simulink model "linearSim"  (R2021b)
settings: Solver=ode23s  StartTime=0.0  StopTime=50  MaxStep=0.01  RelTol=1e-3
undefined symbols (not defined in the file or in its folder): FE, IRL, P, PE, SE
settings Model: Creator=rushik  LastModifiedBy=rushik
settings DataIOCC: SaveOutput=off  DSMLogging=off  SaveTime=off  ReturnWorkspaceOutputs=off

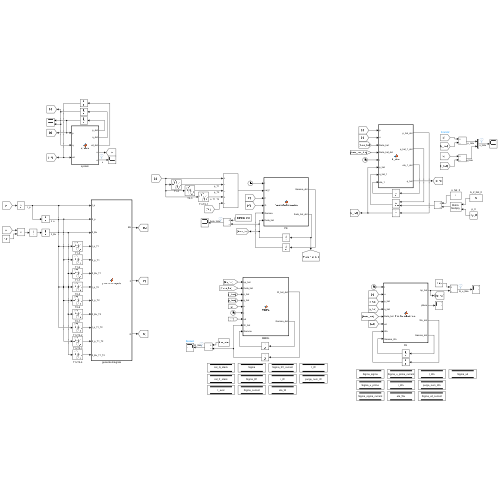
[thumbnail: Simulink's stored preview of the top-level diagram]
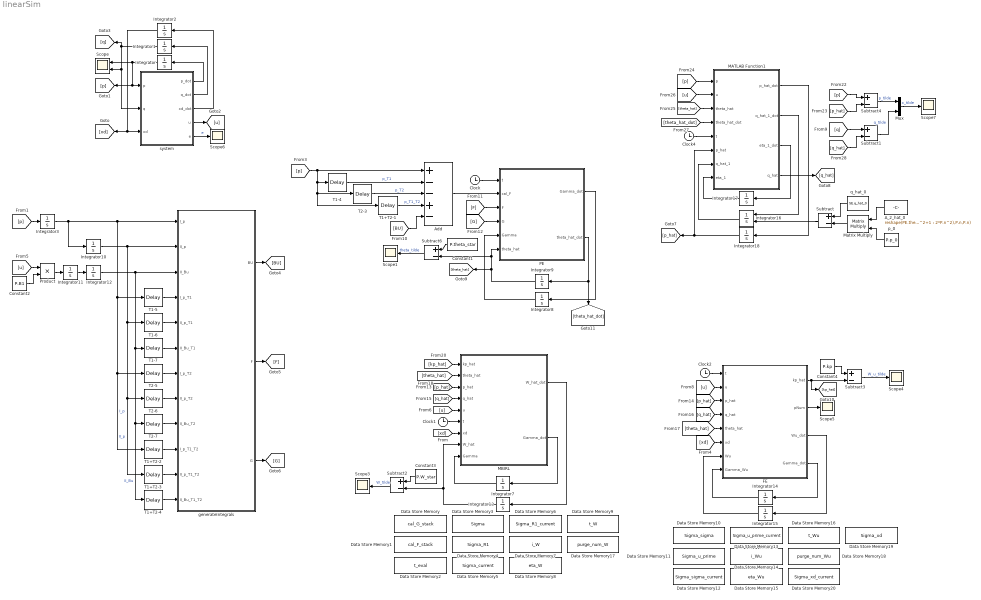
== system linearSim ==
  A_2_hat_0 : Constant  Value=reshape(PE.theta_hat_0(P.n^2+1 : 2*P.n^2),P.n,P.n)
  Add : Sum  Inputs=+--+-
  Clock{,1..2,4} (4 alike) : Clock
  Constant1 : Constant  Value=P.theta_star
  Constant2 : Constant  Value=P.B1
  Constant3 : Constant  Value=P.W_star  VectorParams1D=off
  Constant4 : Constant  Value=P.kp
  Data Store Memory : DataStoreMemory  DataStoreName=cal_G_stack  ReadBeforeWriteMsg=warning  WriteAfterWriteMsg=warning  WriteAfterReadMsg=warning  InitialValue=zeros(2*P.n^2,P.n*PE.N)  VectorParams1D=off  ShowAdditionalParam=off  OutDataTypeStr=double
  Data Store Memory1 : DataStoreMemory  DataStoreName=cal_F_stack  ReadBeforeWriteMsg=warning  WriteAfterWriteMsg=warning  WriteAfterReadMsg=warning  InitialValue=zeros(P.n,PE.N)  VectorParams1D=off  ShowAdditionalParam=off  OutDataTypeStr=double
  Data Store Memory10 : DataStoreMemory  DataStoreName=Sigma_sigma  ReadBeforeWriteMsg=warning  WriteAfterWriteMsg=warning  WriteAfterReadMsg=warning  InitialValue=zeros(FE.M,FE.K)  VectorParams1D=off  ShowAdditionalParam=off  OutDataTypeStr=double
  Data Store Memory11 : DataStoreMemory  DataStoreName=Sigma_u_prime  ReadBeforeWriteMsg=warning  WriteAfterWriteMsg=warning  WriteAfterReadMsg=warning  InitialValue=zeros(FE.M,P.m)  VectorParams1D=off  ShowAdditionalParam=off  OutDataTypeStr=double
  Data Store Memory12 : DataStoreMemory  DataStoreName=Sigma_sigma_current  ReadBeforeWriteMsg=warning  WriteAfterWriteMsg=warning  WriteAfterReadMsg=warning  InitialValue=zeros(FE.M,FE.K)  VectorParams1D=off  ShowAdditionalParam=off  OutDataTypeStr=double
  Data Store Memory13 : DataStoreMemory  DataStoreName=Sigma_u_prime_current  ReadBeforeWriteMsg=warning  WriteAfterWriteMsg=warning  WriteAfterReadMsg=warning  InitialValue=zeros(FE.M,P.m)  VectorParams1D=off  ShowAdditionalParam=off  OutDataTypeStr=double
  Data Store Memory14 : DataStoreMemory  DataStoreName=i_Wu  ReadBeforeWriteMsg=warning  WriteAfterWriteMsg=warning  WriteAfterReadMsg=warning  InitialValue=1  VectorParams1D=off  ShowAdditionalParam=off  OutDataTypeStr=double
  Data Store Memory15 : DataStoreMemory  DataStoreName=eta_Wu  ReadBeforeWriteMsg=warning  WriteAfterWriteMsg=warning  WriteAfterReadMsg=warning  VectorParams1D=off  ShowAdditionalParam=off  OutDataTypeStr=double
  Data Store Memory16 : DataStoreMemory  DataStoreName=t_Wu  ReadBeforeWriteMsg=warning  WriteAfterWriteMsg=warning  WriteAfterReadMsg=warning  VectorParams1D=off  ShowAdditionalParam=off  OutDataTypeStr=double
  Data Store Memory17 : DataStoreMemory  DataStoreName=purge_num_W  ReadBeforeWriteMsg=warning  WriteAfterWriteMsg=warning  WriteAfterReadMsg=warning  VectorParams1D=off  ShowAdditionalParam=off  OutDataTypeStr=double
  Data Store Memory18 : DataStoreMemory  DataStoreName=purge_num_Wu  ReadBeforeWriteMsg=warning  WriteAfterWriteMsg=warning  WriteAfterReadMsg=warning  VectorParams1D=off  ShowAdditionalParam=off  OutDataTypeStr=double
  Data Store Memory19 : DataStoreMemory  DataStoreName=Sigma_xd  ReadBeforeWriteMsg=warning  WriteAfterWriteMsg=warning  WriteAfterReadMsg=warning  InitialValue=zeros(PE.L,FE.M)  VectorParams1D=off  ShowAdditionalParam=off  OutDataTypeStr=double
  Data Store Memory2 : DataStoreMemory  DataStoreName=t_eval  ReadBeforeWriteMsg=warning  WriteAfterWriteMsg=warning  WriteAfterReadMsg=warning  VectorParams1D=off  ShowAdditionalParam=off  OutDataTypeStr=double
  Data Store Memory20 : DataStoreMemory  DataStoreName=Sigma_xd_current  ReadBeforeWriteMsg=warning  WriteAfterWriteMsg=warning  WriteAfterReadMsg=warning  InitialValue=zeros(PE.L,FE.M)  VectorParams1D=off  ShowAdditionalParam=off  OutDataTypeStr=double
  Data Store Memory3 : DataStoreMemory  DataStoreName=Sigma  ReadBeforeWriteMsg=warning  WriteAfterWriteMsg=warning  WriteAfterReadMsg=warning  InitialValue=zeros(2*IRL.N,IRL.num_weights)  VectorParams1D=off  ShowAdditionalParam=off  OutDataTypeStr=double
  Data Store Memory4 : DataStoreMemory  DataStoreName=Sigma_R1  ReadBeforeWriteMsg=warning  WriteAfterWriteMsg=warning  WriteAfterReadMsg=warning  InitialValue=zeros(2*IRL.N,1)  VectorParams1D=off  ShowAdditionalParam=off  OutDataTypeStr=double
  Data Store Memory5 : DataStoreMemory  DataStoreName=Sigma_current  ReadBeforeWriteMsg=warning  WriteAfterWriteMsg=warning  WriteAfterReadMsg=warning  InitialValue=zeros(2*IRL.N,IRL.num_weights)  VectorParams1D=off  ShowAdditionalParam=off  OutDataTypeStr=double
  Data Store Memory6 : DataStoreMemory  DataStoreName=Sigma_R1_current  ReadBeforeWriteMsg=warning  WriteAfterWriteMsg=warning  WriteAfterReadMsg=warning  InitialValue=zeros(2*IRL.N,1)  VectorParams1D=off  ShowAdditionalParam=off  OutDataTypeStr=double
  Data Store Memory7 : DataStoreMemory  DataStoreName=i_W  ReadBeforeWriteMsg=warning  WriteAfterWriteMsg=warning  WriteAfterReadMsg=warning  InitialValue=1  VectorParams1D=off  ShowAdditionalParam=off  OutDataTypeStr=double
  Data Store Memory8 : DataStoreMemory  DataStoreName=eta_W  ReadBeforeWriteMsg=warning  WriteAfterWriteMsg=warning  WriteAfterReadMsg=warning  VectorParams1D=off  ShowAdditionalParam=off  OutDataTypeStr=double
  Data Store Memory9 : DataStoreMemory  DataStoreName=t_W  ReadBeforeWriteMsg=warning  WriteAfterWriteMsg=warning  WriteAfterReadMsg=warning  VectorParams1D=off  ShowAdditionalParam=off  OutDataTypeStr=double
  FE : MATLAB Function  TreatAsAtomicUnit=on
  Integrator : Integrator  InitialCondition=P.p_0
  Integrator1 : Integrator  InitialCondition=P.q_0
  Integrator{3,10..12,17} (5 alike) : Integrator  InitialCondition=zeros(P.n,1)
  Integrator13 : Integrator  InitialCondition=IRL.W_hat_0
  Integrator14 : Integrator  InitialCondition=FE.Gamma_Wu_0
  Integrator15 : Integrator  InitialCondition=FE.Wu_0
  Integrator16 : Integrator  InitialConditionSource=external  InitialCondition=SE.qHat0
  Integrator18 : Integrator  InitialCondition=P.p_0
  Integrator2 : Integrator  InitialCondition=P.x_d_0
  Integrator7 : Integrator  InitialCondition=IRL.Gamma_W_0
  Integrator8 : Integrator  InitialCondition=PE.Gamma_0
  Integrator9 : Integrator  InitialCondition=PE.theta_hat_0
  MATLAB Function1 : MATLAB Function  TreatAsAtomicUnit=on
  MBIRL : MATLAB Function  TreatAsAtomicUnit=on
  Matrix Multiply : Product  Multiplication=Matrix(*)
  Mux : Mux  Inputs=2
  PE : MATLAB Function  TreatAsAtomicUnit=on
  Product : Product
  Scope : Scope  NumInputPorts=2
  Scope{1,3..7} (6 alike) : Scope
  Subtract{,1..4,6} (6 alike) : Sum  Inputs=+-
  T1+T2-{1..4} (4 alike) : TransportDelay  DelayTime=PE.T2 + PE.T1
  T1-{4..7} (4 alike) : TransportDelay  DelayTime=PE.T1
  T2-{3,5..7} (4 alike) : TransportDelay  DelayTime=PE.T2
  generateIntegrals : MATLAB Function  TreatAsAtomicUnit=on
  p_0 : Constant  Value=P.p_0
  q_hat_0 : Constant  Value=SE.q_hat_0
  system : MATLAB Function  TreatAsAtomicUnit=on
  wires:
  system/1(p_dot) -> Integrator/1
  system/2(q_dot) -> Integrator1/1
  system/3(xd_dot) -> Integrator2/1
  Integrator1/1 -> [q], system/2(q), Scope/2
  Integrator2/1 -> [xd], system/3(xd)
  system/4(u) -> [u]
  Integrator3/1 -> Integrator10/1, T1+T2-2/1, T2-5/1, T1-5/1, generateIntegrals/1(I_p)  "I_p"
  Integrator/1 -> Scope/1, [p], system/1(p)
  T1-4/1 -> Add/2  "p_T1"
  T2-3/1 -> Add/3  "p_T2"
  T1+T2-1/1 -> Add/4  "p_T1_T2"
  Add/1 -> PE/2(cal_F)
  PE/1(Gamma_dot) -> Integrator8/1
  Clock/1 -> PE/1(t)
  Integrator8/1 -> PE/5(Gamma)
  PE/2(theta_hat_dot) -> Integrator9/1, [theta_hat_dot]
  Integrator9/1 -> [theta_hat], PE/6(theta_hat), Subtract6/2
  Constant1/1 -> Subtract6/1
  Subtract6/1 -> Scope1/1  "theta_tilde"
  Integrator10/1 -> T1+T2-3/1, T2-6/1, T1-6/1, generateIntegrals/2(II_p)  "II_p"
  Constant2/1 -> Product/2
  Product/1 -> Integrator11/1
  Integrator11/1 -> Integrator12/1
  Integrator12/1 -> T1+T2-4/1, T2-7/1, T1-7/1, generateIntegrals/3(II_Bu)  "II_Bu"
  T1-5/1 -> generateIntegrals/4(I_p_T1)
  T1-6/1 -> generateIntegrals/5(II_p_T1)
  T1-7/1 -> generateIntegrals/6(II_Bu_T1)
  T2-5/1 -> generateIntegrals/7(I_p_T2)
  T2-6/1 -> generateIntegrals/8(II_p_T2)
  T2-7/1 -> generateIntegrals/9(II_Bu_T2)
  T1+T2-2/1 -> generateIntegrals/10(I_p_T1_T2)
  T1+T2-3/1 -> generateIntegrals/11(II_p_T1_T2)
  T1+T2-4/1 -> generateIntegrals/12(II_Bu_T1_T2)
  generateIntegrals/1(BU) -> [BU]
  generateIntegrals/2(F) -> [F]
  Subtract1/1 -> Mux/2  "q_tilde"
  MBIRL/2(Gamma_dot) -> Integrator7/1
  Integrator7/1 -> MBIRL/9(Gamma)
  MBIRL/1(W_hat_dot) -> Integrator13/1
  Integrator13/1 -> MBIRL/8(W_hat), Subtract2/2
  Subtract2/1 -> Scope3/1  "W_tilde"
  Constant3/1 -> Subtract2/1
  FE/4(Gamma_dot) -> Integrator14/1
  Integrator14/1 -> FE/8(Gamma_Wu)
  FE/3(Wu_dot) -> Integrator15/1
  Integrator15/1 -> FE/7(Wu)
  FE/1(kp_hat) -> Subtract3/2, [kp_hat]
  Subtract3/1 -> Scope4/1  "W_u_tilde"
  Constant4/1 -> Subtract3/1
  FE/2(pNum) -> Scope5/1
  [p] -> Integrator3/1
  [p] -> T1+T2-1/1, T2-3/1, T1-4/1, Add/1
  [xd] -> MBIRL/7(xd)
  [xd] -> FE/6(xd)
  [u] -> Product/1
  [u] -> MBIRL/5(u)
  [u] -> FE/2(u)
  [q] -> Subtract1/1
  [BU] -> Add/5
  [F] -> PE/3(F)
  generateIntegrals/3(G) -> [G]
  [G] -> PE/4(G)
  Clock1/1 -> MBIRL/6(t)
  Clock2/1 -> FE/1(t)
  [p_hat] -> MBIRL/3(p_hat)
  [p_hat] -> FE/3(p_hat)
  [q_hat] -> MBIRL/4(q_hat)
  [q_hat] -> FE/4(q_hat)
  [theta_hat] -> FE/5(theta_hat)
  [theta_hat] -> MBIRL/2(theta_hat)
  [kp_hat] -> MBIRL/1(kp_hat)
  system/5(e) -> Scope6/1  "e"
  [p] -> Subtract4/1
  [p_hat] -> Subtract4/2
  Subtract4/1 -> Mux/1  "p_tilde"
  Mux/1 -> Scope7/1  "x_tilde"
  A_2_hat_0/1 -> Matrix Multiply/1
  p_0/1 -> Matrix Multiply/2
  Matrix Multiply/1 -> Subtract/2
  q_hat_0/1 -> Subtract/1
  Subtract/1 -> Integrator16/2
  [theta_hat] -> MATLAB Function1/3(theta_hat)
  [p] -> MATLAB Function1/1(p)
  Clock4/1 -> MATLAB Function1/5(t)
  MATLAB Function1/2(q_hat_1_dot) -> Integrator16/1
  [u] -> MATLAB Function1/2(u)
  MATLAB Function1/3(eta_1_dot) -> Integrator17/1
  MATLAB Function1/1(p_hat_dot) -> Integrator18/1
  Integrator18/1 -> [p_hat], MATLAB Function1/6(p_hat)
  Integrator16/1 -> MATLAB Function1/7(q_hat_1)
  Integrator17/1 -> MATLAB Function1/8(eta_1)
  [theta_hat_dot] -> MATLAB Function1/4(theta_hat_dot)
  MATLAB Function1/4(q_hat) -> [q_hat]
  [q_hat] -> Subtract1/2

== matlab function linearSim/FE ==
  settings: updateMethod=DISCRETE
  data: kp_hat output; pNum output; t input; u input; p_hat input; q_hat input; theta_hat input; xd input; Wu_dot output; Wu input; Gamma_Wu input; P parameter; Gamma_dot output; FE parameter; Sigma_sigma data_store_memory; Sigma_u_prime data_store_memory; Sigma_sigma_current data_store_memory; Sigma_u_prime_current data_store_memory; i_Wu data_store_memory; eta_Wu data_store_memory; purge_num_Wu data_store_memory; t_Wu data_store_memory; Sigma_xd data_store_memory; Sigma_xd_current data_store_memory; PE parameter
function [kp_hat,pNum,Wu_dot,Gamma_dot] = FeedbackEstimator(t,u,p_hat,q_hat,theta_hat,xd,Wu,Gamma_Wu,P,FE,PE)

global Sigma_sigma Sigma_u_prime Sigma_sigma_current Sigma_u_prime_current i_Wu eta_Wu purge_num_Wu t_Wu Sigma_xd Sigma_xd_current
if purge_num_Wu == 0
    Wu_dot = zeros(FE.K,P.m);
    Gamma_dot = zeros(FE.K,FE.K);
else
    UD_hat = -[theta_hat(1)+2, theta_hat(2)]*Sigma_xd_current;
    Sigma_u_current = Sigma_u_prime_current - UD_hat.';
    Wu_dot = FE.alpha_u*Gamma_Wu*Sigma_sigma_current'*(-Sigma_u_current-Sigma_sigma_current*Wu);
    Gamma_dot = FE.beta_u*Gamma_Wu - FE.alpha_u*Gamma_Wu*(Sigma_sigma_current.'*Sigma_sigma_current)*Gamma_Wu;
end
pNum = purge_num_Wu;
kp_hat = Wu.';
if t - t_Wu >= FE.t_step
    
    % mu_hat = u - ud_hat;
    e_hat = [p_hat;q_hat]-xd;
    new_SST = Sigma_sigma.'*Sigma_sigma;
    SST = Sigma_sigma_current.'*Sigma_sigma_current;
    eig_Sigma_sigma_new = min(real(eig(new_SST)));
    eig_Sigma_sigma = min(real(eig(SST)));
    
    if eig_Sigma_sigma_new > max(0.5*eig_Sigma_sigma,1e-8) && (t-eta_Wu > FE.tau || purge_num_Wu == 0) && i_Wu >= FE.M
        Sigma_sigma_current = Sigma_sigma;
        Sigma_u_prime_current = Sigma_u_prime;
        Sigma_xd_current = Sigma_xd;
        Sigma_sigma = zeros(FE.M,FE.K);
        Sigma_u_prime = zeros(FE.M,P.m);
        Sigma_xd = zeros(PE.L,FE.M);% need 3D matrix if P.m > 1
        eta_Wu = t;
        i_Wu = 0;
        purge_num_Wu = purge_num_Wu + 1;
    end
    
    eig_list = zeros(FE.M,1);
    for i=1:FE.M
        ith_sigma_sigma = (Sigma_sigma(i,:));
        eig_list(i,1) = min(real(eig(new_SST + e_hat*e_hat.' - ith_sigma_sigma.'*ith_sigma_sigma)));
    end
    [eig_after_replacement,ind]=max(eig_list);
    if eig_after_replacement > eig_Sigma_sigma_new
        Sigma_sigma(ind,:) = e_hat.';
        Sigma_u_prime(ind,:) = u;
        Sigma_xd(:,ind) = xd;
        i_Wu = i_Wu + 1;
    end
    t_Wu = t;
end
end

== matlab function linearSim/MATLAB Function1 ==
  data: p input; u input; theta_hat input; theta_hat_dot input; t input; p_hat input; q_hat_1 input; eta_1 input; p_hat_dot output; q_hat_1_dot output; eta_1_dot output; P parameter; SE parameter; q_hat output
function [p_hat_dot,q_hat_1_dot,eta_1_dot,q_hat] = R_filter(p,u,theta_hat,theta_hat_dot,t,p_hat,q_hat_1,eta_1,P,SE)
    p_tilde = p - p_hat;
    
    A1_hat = reshape(theta_hat(1 : P.n^2),P.n,P.n);
    A2_hat = reshape(theta_hat(P.n^2+1 : 2*P.n^2),P.n,P.n);
    A2_hat_dot = reshape(theta_hat_dot(P.n^2+1 : 2*P.n^2),P.n,P.n);

    p_hat_dot = q_hat_1 + A2_hat*p_hat;
    q_hat_1_dot = (A1_hat - A2_hat_dot)*p + P.B1*u + SE.alpha^2*p_tilde - (SE.k+SE.alpha+SE.beta)*eta_1 + (SE.k+SE.alpha)*(SE.k+SE.alpha+SE.beta)*p_tilde;
    eta_1_dot = -(SE.k+SE.beta)*eta_1 + ((SE.k+SE.beta)*(SE.k+SE.alpha)-SE.k*SE.alpha)*p_tilde;
    
    q_hat = q_hat_1 + A2_hat*p_hat;
end

== matlab function linearSim/PE ==
  settings: updateMethod=DISCRETE
  data: t input; Gamma_dot output; cal_F input; F input; G input; Gamma input; theta_hat input; theta_hat_dot output; P parameter; PE parameter; cal_G_stack data_store_memory; cal_F_stack data_store_memory; t_eval data_store_memory
function [Gamma_dot,theta_hat_dot]  = ParameterEstimation(t,cal_F,F,G,Gamma,theta_hat,P,PE)
%#codegen

global cal_F_stack cal_G_stack t_eval;

cal_G = [kron(F,eye(P.n)).' kron(G,eye(P.n)).'];

if t - t_eval >= PE.t_step && t >= PE.T1 + PE.T2
    current_script_G = cal_G_stack*cal_G_stack';
    current_singular_value = min(svd(current_script_G));
    singular_value_list = zeros(PE.N,1);
    for i=1:PE.N
        ith_cal_G_transpose = cal_G_stack(:,(i-1)*P.n+1:i*P.n);
        new_script_G = current_script_G + cal_G'*cal_G...
            -ith_cal_G_transpose*ith_cal_G_transpose';
        singular_value_list(i,1)=min(svd(new_script_G));
    end
    [new_singular_value,max_index]=max(singular_value_list);
    
    if new_singular_value>=current_singular_value
        cal_G_stack(:,(max_index-1)*P.n+1:max_index*P.n) = cal_G';
        cal_F_stack(:,max_index) = cal_F;
    end
    t_eval = t;
end

theta_hat_dot = PE.k_theta*Gamma*(cal_G_stack*...
    (reshape(cal_F_stack,P.n*PE.N,1)-cal_G_stack'*theta_hat));
    
Gamma_dot = PE.beta*Gamma - PE.k_theta*Gamma*...
    (cal_G_stack*cal_G_stack')*Gamma- PE.k_theta*Gamma*...
    (cal_G'*cal_G)*Gamma;
end

== matlab function linearSim/generateIntegrals ==
  data: BU output; I_p input; F output; II_p input; II_Bu input; I_p_T1 input; II_p_T1 input; II_Bu_T1 input; I_p_T2 input; II_p_T2 input; II_Bu_T2 input; I_p_T1_T2 input; II_p_T1_T2 input; II_Bu_T1_T2 input; G output
function [BU, F, G] = generateIntegrals(I_p,II_p,II_Bu,I_p_T1,II_p_T1,II_Bu_T1,I_p_T2,II_p_T2,II_Bu_T2,I_p_T1_T2,II_p_T1_T2,II_Bu_T1_T2)

F = II_p - II_p_T1 - II_p_T2 + II_p_T1_T2;

G = I_p - I_p_T1 - I_p_T2 + I_p_T1_T2;

BU = II_Bu - II_Bu_T1 - II_Bu_T2 + II_Bu_T1_T2;

end

== matlab function linearSim/system ==
  data: p input; p_dot output; q input; xd input; q_dot output; xd_dot output; P parameter; u output; e output
function [p_dot,q_dot,xd_dot,u,e] = system(p,q,xd,P)
    x = [p;q];
    ud = P.B_plus*(P.Ad - P.A)*xd;
    e=(x-xd);
    mu = -P.kp*e;
    u = mu + ud;

    p_dot = q;
    q_dot = P.A1*p + P.A2*q + P.B1*u;
    xd_dot = P.Ad*xd;
end

== matlab function linearSim/MBIRL ==
  settings: updateMethod=DISCRETE
  data: kp_hat input; theta_hat input; p_hat input; q_hat input; u input; t input; xd input; W_hat input; P parameter; W_hat_dot output; Gamma_dot output; IRL parameter; t_W data_store_memory; Sigma data_store_memory; Sigma_R1 data_store_memory; Sigma_R1_current data_store_memory; Sigma_current data_store_memory; i_W data_store_memory; eta_W data_store_memory; Gamma input; purge_num_W data_store_memory
function [W_hat_dot,Gamma_dot] =...
    MBIRL(kp_hat,theta_hat,p_hat,q_hat,u,t,xd,W_hat,P,IRL,Gamma)


global Sigma Sigma_R1 Sigma_current Sigma_R1_current i_W eta_W t_W purge_num_W

ud_hat = -[theta_hat(1)+2, theta_hat(2)]*xd;
if IRL.feedback_driven
    e = -IRL.max_e + 2*IRL.max_e.*rand(2,1);
    mu = -kp_hat*(e);
else
    x_hat = [p_hat;q_hat];
    mu = u - ud_hat;
    e = x_hat-xd;
end

e1 = e(1);
e2 = e(2);

grad_x_sigma_V= [[ 2*e1,    0];
                [     0, 2*e2];
                [    e2,   e1]];

IRL_theta_hat = [[0;0] theta_hat];
sigma = e;
f_o = [e2;0] + P.B*mu;
Y_hat = f_o + IRL_theta_hat.'*sigma;

sigma_Q_hat = [e1^2;e2^2];
sigma_R1_minus = [];
sigma_double_prime = [grad_x_sigma_V*Y_hat;sigma_Q_hat;sigma_R1_minus];

grad_u_f_o = P.B;
grad_u_sigma = zeros(size(sigma));
G = grad_u_f_o.'*grad_x_sigma_V.' + (IRL_theta_hat.'*grad_u_sigma).'*grad_x_sigma_V.';
sigma_R2_minus = [];
sigma_triple_prime = [sigma_double_prime [G.';zeros(size(sigma_Q_hat));2*sigma_R2_minus.']];
sigma_R1 = [P.R(1,1)*mu^2;2*P.R(1,1)*mu];

if purge_num_W == 0
    W_hat_dot = zeros(IRL.num_weights,1);
    Gamma_dot = zeros(IRL.num_weights,IRL.num_weights);
else
    W_hat_dot = IRL.alpha*Gamma*Sigma_current'*(-Sigma_current*W_hat+Sigma_R1_current);
    Gamma_dot = IRL.beta*Gamma - IRL.alpha*Gamma*(Sigma_current'*Sigma_current)*Gamma;
end

if t - t_W >= IRL.t_step
    if i_W <= IRL.N
        Sigma(2*i_W-1:2*i_W,:) = sigma_triple_prime.';
        Sigma_R1(2*i_W-1:2*i_W,:) = -sigma_R1;
        i_W = i_W + 1;
        eta_W = t;
    else
        new_SST = Sigma.'*Sigma;
        new_con_num = cond(new_SST);
        con_num_list = zeros(IRL.N,1);
        for i=1:IRL.N
            ith_sigma = Sigma(2*i-1:2*i,:);
            new_SST = new_SST + sigma_triple_prime*sigma_triple_prime.'...
                -ith_sigma.'*ith_sigma;
            con_num_list(i,1)=cond(new_SST);
        end
        [c_num_aft_rep,ind]=min(con_num_list);
        if c_num_aft_rep < new_con_num
            Sigma(2*ind-1:2*ind,:) = sigma_triple_prime.';
            Sigma_R1(2*ind-1:2*ind,:) = -sigma_R1;
            new_con_num = c_num_aft_rep;
        end
        if new_con_num < 1e20
            Sigma_current = Sigma;
            Sigma_R1_current = Sigma_R1;
            if abs(eta_W-t) > IRL.tau
               Sigma = zeros(2*IRL.N,IRL.num_weights);
               Sigma_R1 = zeros(2*IRL.N,1);
               i_W=1;
               eta_W=t;
               purge_num_W = purge_num_W + 1;
            end
        end
    end
    t_W = t;
end
end
